simulink model "Q5_factorization"  (R2021b)
settings: Solver=ode45  StartTime=0.0  StopTime=5  RelTol=1e-3  EnableMultiTasking=on
undefined symbols (not defined in the file or in its folder): H_x, H_y
libraries: cstblocks x20
settings Model: Creator=Admin  LastModifiedBy=user
settings SolverCC: AlgebraicLoopSolver=TrustRegion
settings DataIOCC: LimitDataPoints=on  SaveFormat=Array  ReturnWorkspaceOutputs=off
settings OptimizationCC: ExpressionDepthLimit=2147483647  LifeSpan=inf
settings DebuggingCC: UnderspecifiedInitializationDetection=Classic  MergeDetectMultiDrivingBlocksExec=none  SolverPrmCheckMsg=warning  StateNameClashWarn=warning  SFUnexpectedBacktrackingDiag=warning  SFNoUnconditionalDefaultTransitionDiag=warning  SFExecutionAtInitializationDiag=none  SFMachineParentedDataDiag=warning  ArithmeticOperatorsInVariantConditions=warning
settings HardwareCC: ProdBitPerPointer=32  ProdBitPerSizeT=32  ProdBitPerPtrDiffT=32  ProdLargestAtomicFloat=None  ProdIntDivRoundTo=Undefined  ProdEndianess=Unspecified  ProdWordSize=32  ProdHWDeviceType=32-bit Generic
settings ModelReferenceCC: PropagateSignalLabelsOutOfModel=off
settings SFSimCC: SimUseLocalCustomCode=off  CustomCodeUndefinedFunction=UseInterfaceOnly
settings RTWCC: RTWUseLocalCustomCode=off
settings CodeAppCC: StateflowObjectComments=on
settings GRTTargetCC: TargetLangStandard=C89/C90 (ANSI)
settings ConfigComp: CovMetricSettings=dw  CovSaveCumulativeToWorkspaceVar=on  CovSaveSingleToWorkspaceVar=on  CovExternalEMLEnable=off

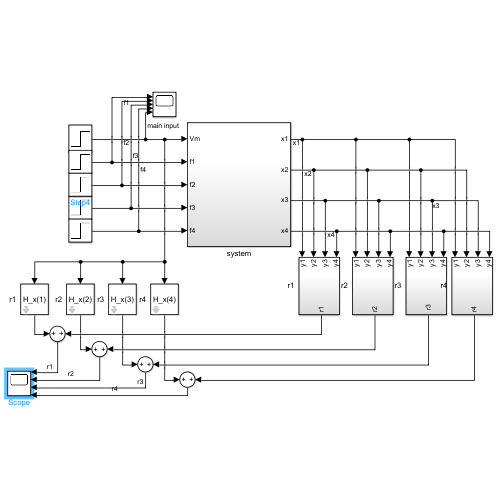
[thumbnail: Simulink's stored preview of the top-level diagram]
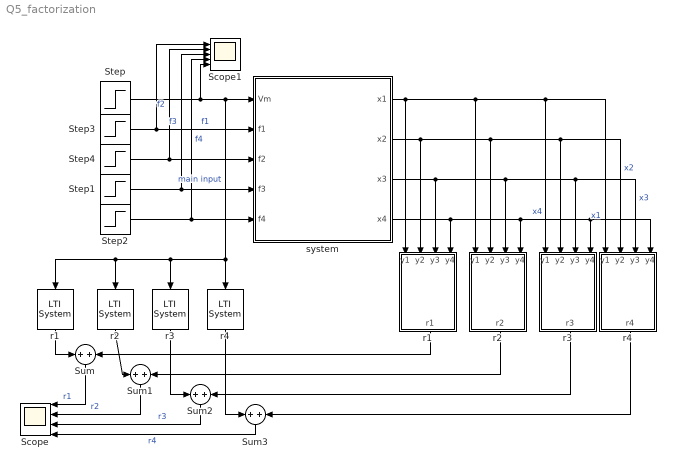
== system Q5_factorization ==
  " r1" : Subsystem
  " r2" : Subsystem
  " r3" : cstblocks/LTI System  sys=H_x(3)  IC=[]
  " r4" : cstblocks/LTI System  sys=H_x(4)  IC=[]
  Scope : Scope  NumInputPorts=4
  Scope1 : Scope  NumInputPorts=5
  Step{,1,3..4} (4 alike) : Step  Time=0  After=0  SampleTime=0
  Step2 : Step  Time=2  After=2  SampleTime=0
  Sum{,1..3} (4 alike) : Sum
  r1 : cstblocks/LTI System  sys=H_x(1)  IC=[]
  r2 : cstblocks/LTI System  sys=H_x(2)  IC=[]
  r3 : Subsystem
  r4 : Subsystem
  system : Subsystem
  wires:
  Step/1 -> Scope1/5, system/1(Vm), r1/1, r2/1, " r3"/1, " r4"/1  "main input"
  system/1(x1) -> r4/1(y1), r3/1(y1), " r2"/1(y1), " r1"/1(y1)  "x1"
  system/2(x2) -> r4/2(y2), r3/2(y2), " r2"/2(y2), " r1"/2(y2)  "x2"
  system/4(x4) -> r4/4(y4), r3/4(y4), " r2"/4(y4), " r1"/4(y4)  "x4"
  r1/1 -> Sum/1
  r2/1 -> Sum1/1
  " r3"/1 -> Sum2/1
  " r4"/1 -> Sum3/1
  " r1"/1(r1) -> Sum/2
  system/3(x3) -> " r1"/3(y3), " r2"/3(y3), r3/3(y3), r4/3(y3)  "x3"
  " r2"/1(r2) -> Sum1/2
  r3/1(" r3 ") -> Sum2/2
  r4/1("r4 ") -> Sum3/2
  Sum/1 -> Scope/1  "r1"
  Sum1/1 -> Scope/2  "r2"
  Sum2/1 -> Scope/3  "r3"
  Sum3/1 -> Scope/4  "r4"
  Step1/1 -> Scope1/3, system/4(f3)  "f3"
  Step2/1 -> Scope1/4, system/5("f4 ")  "f4"
  Step4/1 -> Scope1/2, system/3(f2)  "f2"
  Step3/1 -> Scope1/1, system/2(f1)  "f1"

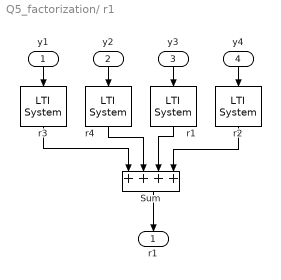
== system Q5_factorization/ r1 ==
  y1 : Inport
  y2 : Inport  Port=2
  y3 : Inport  Port=3
  y4 : Inport  Port=4
  " r1" : cstblocks/LTI System  sys=H_y(1,3)  IC=[]
  " r2" : cstblocks/LTI System  sys=H_y(1,4)  IC=[]
  Sum : Sum  Inputs=++++
  r3 : cstblocks/LTI System  sys=H_y(1,1)  IC=[]
  r4 : cstblocks/LTI System  sys=H_y(1,2)  IC=[]
  r1 : Outport
  wires:
  y2/1 -> r4/1
  y1/1 -> r3/1
  y4/1 -> " r2"/1
  y3/1 -> " r1"/1
  r3/1 -> Sum/1
  r4/1 -> Sum/2
  " r1"/1 -> Sum/3
  " r2"/1 -> Sum/4
  Sum/1 -> r1/1

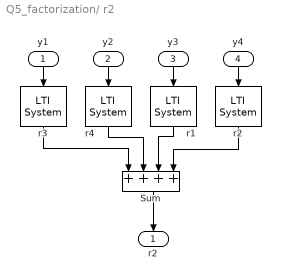
== system Q5_factorization/ r2 ==
  y1 : Inport
  y2 : Inport  Port=2
  y3 : Inport  Port=3
  y4 : Inport  Port=4
  " r1" : cstblocks/LTI System  sys=H_y(2,3)  IC=[]
  " r2" : cstblocks/LTI System  sys=H_y(2,4)  IC=[]
  Sum : Sum  Inputs=++++
  r3 : cstblocks/LTI System  sys=H_y(2,1)  IC=[]
  r4 : cstblocks/LTI System  sys=H_y(2,2)  IC=[]
  r2 : Outport
  wires:
  Sum/1 -> r2/1
  " r2"/1 -> Sum/4
  " r1"/1 -> Sum/3
  r4/1 -> Sum/2
  r3/1 -> Sum/1
  y3/1 -> " r1"/1
  y4/1 -> " r2"/1
  y1/1 -> r3/1
  y2/1 -> r4/1

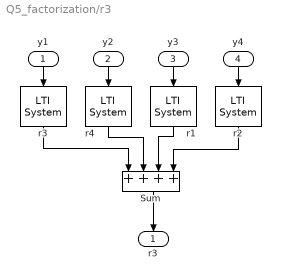
== system Q5_factorization/r3 ==
  y1 : Inport
  y2 : Inport  Port=2
  y3 : Inport  Port=3
  y4 : Inport  Port=4
  " r1" : cstblocks/LTI System  sys=H_y(3,3)  IC=[]
  " r2" : cstblocks/LTI System  sys=H_y(3,4)  IC=[]
  Sum : Sum  Inputs=++++
  r3 : cstblocks/LTI System  sys=H_y(3,1)  IC=[]
  r4 : cstblocks/LTI System  sys=H_y(3,2)  IC=[]
  " r3 " : Outport
  wires:
  y2/1 -> r4/1
  y1/1 -> r3/1
  y4/1 -> " r2"/1
  y3/1 -> " r1"/1
  r3/1 -> Sum/1
  r4/1 -> Sum/2
  " r1"/1 -> Sum/3
  " r2"/1 -> Sum/4
  Sum/1 -> " r3 "/1

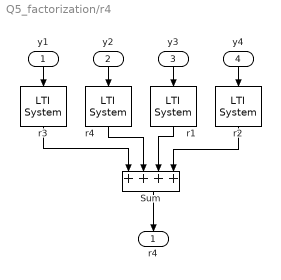
== system Q5_factorization/r4 ==
  y1 : Inport
  y2 : Inport  Port=2
  y3 : Inport  Port=3
  y4 : Inport  Port=4
  " r1" : cstblocks/LTI System  sys=H_y(4,3)  IC=[]
  " r2" : cstblocks/LTI System  sys=H_y(4,4)  IC=[]
  Sum : Sum  Inputs=++++
  r3 : cstblocks/LTI System  sys=H_y(4,1)  IC=[]
  r4 : cstblocks/LTI System  sys=H_y(4,2)  IC=[]
  "r4 " : Outport
  wires:
  Sum/1 -> "r4 "/1
  " r2"/1 -> Sum/4
  " r1"/1 -> Sum/3
  r4/1 -> Sum/2
  r3/1 -> Sum/1
  y3/1 -> " r1"/1
  y4/1 -> " r2"/1
  y1/1 -> r3/1
  y2/1 -> r4/1

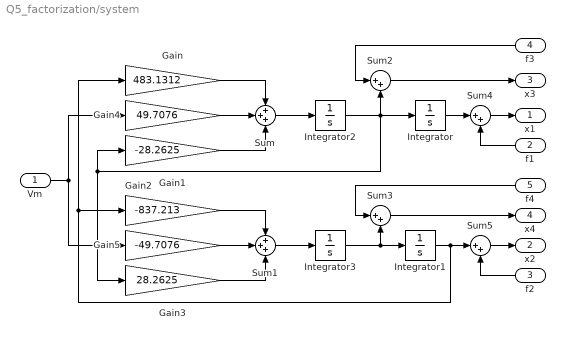
== system Q5_factorization/system ==
  Vm : Inport
  f1 : Inport  Port=2
  f2 : Inport  Port=3
  f3 : Inport  Port=4
  "f4 " : Inport  Port=5
  Gain : Gain  Gain=483.1312
  Gain1 : Gain  Gain=-28.2625
  Gain2 : Gain  Gain=-837.213
  Gain3 : Gain  Gain=28.2625
  Gain4 : Gain  Gain=49.7076
  Gain5 : Gain  Gain=-49.7076
  Integrator{,1..3} (4 alike) : Integrator
  Sum : Sum  Inputs=+++
  Sum1 : Sum  Inputs=+++
  Sum{2..5} (4 alike) : Sum  Inputs=|++
  x1 : Outport
  x2 : Outport  Port=2
  x3 : Outport  Port=3
  x4 : Outport  Port=4
  wires:
  Gain1/1 -> Sum/3
  Integrator1/1 -> Sum5/1, Gain/1, Gain2/1
  Integrator2/1 -> Sum2/2, Integrator/1, Gain3/1, Gain1/1
  Gain/1 -> Sum/1
  Gain5/1 -> Sum1/2
  Sum/1 -> Integrator2/1
  Sum1/1 -> Integrator3/1
  Gain2/1 -> Sum1/1
  Gain3/1 -> Sum1/3
  Gain4/1 -> Sum/2
  Vm/1 -> Gain4/1, Gain5/1
  Integrator3/1 -> Integrator1/1, Sum3/2
  Sum2/1 -> x3/1
  Sum3/1 -> x4/1
  Integrator/1 -> Sum4/1
  Sum4/1 -> x1/1
  Sum5/1 -> x2/1
  f3/1 -> Sum2/1
  "f4 "/1 -> Sum3/1
  f1/1 -> Sum4/2
  f2/1 -> Sum5/2
